simulink model "Test_CAN_Communication"  (R2015b)
settings: Solver=VariableStepAuto  StartTime=0.0  StopTime=10.0  RelTol=1e-3
undefined symbols (not defined in the file): canChannel
libraries: canlib x5, canmsglib x4, simulink x1
settings Model: Creator=Alexander  LastModifiedBy=Alexander

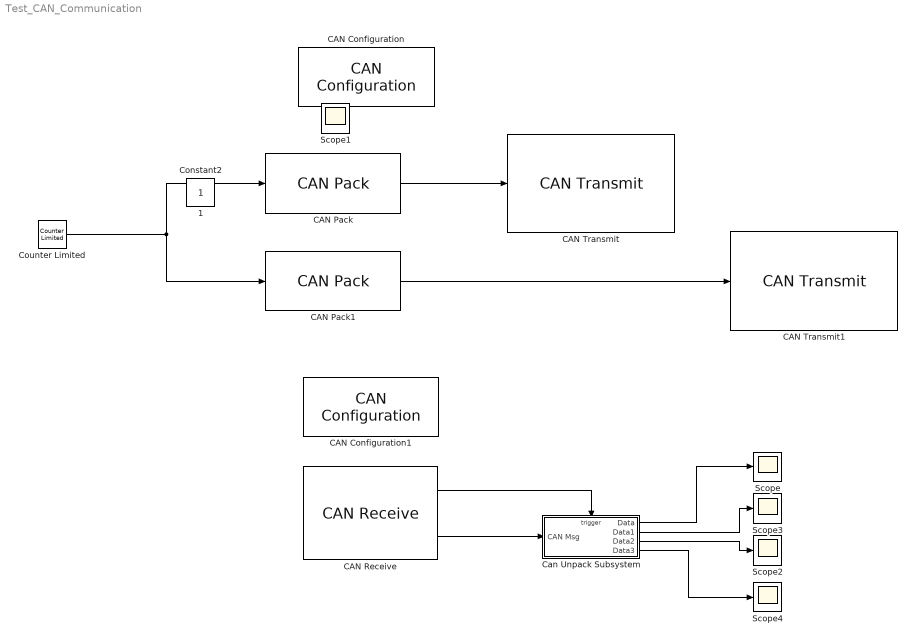
== system Test_CAN_Communication ==
  CAN Configuration : canlib/CAN Configuration  BlockHandle=1938.0004  DeviceMenu=Kvaser Virtual 1 (Channel 1)  Device=Kvaser Virtual 1 (Channel 1)  ObjConstructor=canChannel('Kvaser', 'Virtual 1', 1)  BusSpeed=500000  EnableBitParameters=off  SJW=1  TSEG1=4  TSEG2=3  NSamples=1  AckMode=Normal
  CAN Configuration1 : canlib/CAN Configuration  BlockHandle=1939.0004  DeviceMenu=Kvaser Virtual 1 (Channel 2)  Device=Kvaser Virtual 1 (Channel 2)  ObjConstructor=canChannel('Kvaser', 'Virtual 1', 2)  BusSpeed=500000  EnableBitParameters=off  SJW=1  TSEG1=4  TSEG2=3  NSamples=1  AckMode=Normal
  CAN Pack : canmsglib/CAN Pack  MsgList=(none)  MsgName=CAN Msg  MsgIDType=Standard (11-bit identifier)  MsgIdentifier=250  MsgLength=8  NSignals=0  StartBits=0  SignalSizes=0  ByteOrders=0  DataTypes=0  MultiplexTypes=0  MultiplexValues=0  Factors=0  Offsets=0  Minimums=0  Maximums=0  Remote=off
      settings: DataFormat=raw data
  CAN Pack1 : canmsglib/CAN Pack  MsgList=(none)  MsgName=CAN Msg  MsgIDType=Standard (11-bit identifier)  MsgIdentifier=500  MsgLength=8  NSignals=0  StartBits=0  SignalSizes=0  ByteOrders=0  DataTypes=0  MultiplexTypes=0  MultiplexValues=0  Factors=0  Offsets=0  Minimums=0  Maximums=0  Remote=off
      settings: DataFormat=raw data
  CAN Receive : canlib/CAN Receive  BlockHandle=1941.0004  DeviceMenu=Kvaser Virtual 1 (Channel 2)  Device=Kvaser Virtual 1 (Channel 2)  ObjConstructor=canChannel('Kvaser', 'Virtual 1', 2)  EnableStandardIDsFilter=off  StandardIDs=[250 500]  EnableExtendedIDsFilter=off  ExtendedIDs=0  SampleTime=0.01  MsgsPerTimestep=all  StdIDsCombo=Allow only  ExtIDsCombo=Allow all  InternalFilterUpdateStatus=on
  CAN Transmit : canlib/CAN Transmit  BlockHandle=1942.0004  DeviceMenu=Kvaser Virtual 1 (Channel 1)  Device=Kvaser Virtual 1 (Channel 1)  ObjConstructor=canChannel('Kvaser', 'Virtual 1', 1)  EnablePeriodicTransmit=on  MessagePeriod=1.000
  CAN Transmit1 : canlib/CAN Transmit  BlockHandle=2016.0006  DeviceMenu=Kvaser Virtual 1 (Channel 1)  Device=Kvaser Virtual 1 (Channel 1)  ObjConstructor=canChannel('Kvaser', 'Virtual 1', 1)  EnablePeriodicTransmit=on  MessagePeriod=0.500
  Can Unpack Subsystem : Subsystem  TreatAsAtomicUnit=on
  Counter Limited : simulink/Sources/Counter Limited  uplimit=50  tsamp=0.01
  Scope{,1..4} (5 alike) : Scope
  1 : Constant  IOType=siggen
  Constant2 : Constant  IOType=siggen
  wires:
  Can Unpack Subsystem/1(Data) -> Scope/1
  CAN Receive/2 -> Can Unpack Subsystem/1(CAN Msg)
  CAN Receive/1 -> Can Unpack Subsystem/Trigger
  Counter Limited/1 -> CAN Pack1/1, CAN Pack/1
  CAN Pack1/1 -> CAN Transmit1/1
  CAN Pack/1 -> CAN Transmit/1
  Can Unpack Subsystem/2(Data1) -> Scope3/1
  Can Unpack Subsystem/3(Data2) -> Scope2/1
  Can Unpack Subsystem/4(Data3) -> Scope4/1

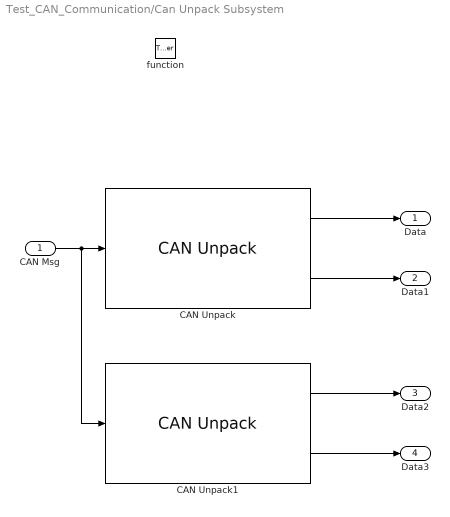
== system Test_CAN_Communication/Can Unpack Subsystem ==
  CAN Msg : Inport
  function : TriggerPort  TriggerType=function-call
  CAN Unpack : canmsglib/CAN Unpack  MsgList=(none)  MsgName=CAN Msg  MsgIDType=Standard (11-bit identifier)  MsgIdentifier=250  MsgLength=1  NSignals=0  IDPort=off  TimestampPort=on  ErrorPort=off  RemotePort=off  LengthPort=off  StatusPort=off  StartBits=0  SignalSizes=0  ByteOrders=0  DataTypes=0  MultiplexTypes=0  MultiplexValues=0  Factors=0  Offsets=0  Minimums=0  Maximums=0
      settings: DataFormat=raw data
  CAN Unpack1 : canmsglib/CAN Unpack  MsgList=(none)  MsgName=CAN Msg  MsgIDType=Standard (11-bit identifier)  MsgIdentifier=500  MsgLength=1  NSignals=0  IDPort=off  TimestampPort=on  ErrorPort=off  RemotePort=off  LengthPort=off  StatusPort=off  StartBits=0  SignalSizes=0  ByteOrders=0  DataTypes=0  MultiplexTypes=0  MultiplexValues=0  Factors=0  Offsets=0  Minimums=0  Maximums=0
      settings: DataFormat=raw data
  Data : Outport
  Data1 : Outport  Port=2
  Data2 : Outport  Port=3
  Data3 : Outport  Port=4
  wires:
  CAN Unpack/1 -> Data/1
  CAN Msg/1 -> CAN Unpack1/1, CAN Unpack/1
  CAN Unpack/2 -> Data1/1
  CAN Unpack1/1 -> Data2/1
  CAN Unpack1/2 -> Data3/1
